simulink model "DIPC4M"  (R2015a)
settings: Solver=ode3  SolverMode=SingleTasking  StartTime=0.0  StopTime=3  FixedStep=1e-3  RelTol=1e-7
values from neighbouring files (symbols this model uses):
  alpha = 1.5    [CaViInit.m]    (also in CaccavaleVillani.m = 2)
  d1 = 1000    [CaViInit.m]    (also in CaccavaleVillani.m = 100)
  delta1 = 80    [CaViInit.m]    (also in CaccavaleVillani.m = 100)
  deltao = 10    [CaViInit.m]    (also in CaccavaleVillani.m = 2000)
  Do = 1500    [CaViInit.m]    (also in CaccavaleVillani.m = 2000)
  g = [0;0;-9.81]    [CaViInit.m]    (also in CaccavaleVillani.m)
  j0 = 0.2    [CaViInit.m]    (also in CaccavaleVillani.m = 1)
  j1 = 2    [CaViInit.m]    (also in CaccavaleVillani.m = 1)
  j1d = 1.00*j1    (= 2)    [CaViInit.m]    (also in CaccavaleVillani.m = 1)
  j2 = 2    [CaViInit.m]    (also in CaccavaleVillani.m = 1)
  j2d = 1.00*j2    (= 2)    [CaViInit.m]    (also in CaccavaleVillani.m = 1)
  j3 = 2    [CaViInit.m]    (also in CaccavaleVillani.m = 1)
  j3d = 1.00*j3    (= 2)    [CaViInit.m]    (also in CaccavaleVillani.m = 1)
  j4 = 2    [CaViInit.m]    (also in CaccavaleVillani.m = 1)
  j4d = 1.00*j4    (= 2)    [CaViInit.m]    (also in CaccavaleVillani.m = 1)
  k1 = 400    [CaViInit.m]    (also in CaccavaleVillani.m = 10000)
  K_o = 700    [CaViInit.m]    (also in CaccavaleVillani.m = 10000)
  kappa1 = 2    [CaViInit.m]    (also in CaccavaleVillani.m = 250)
  kappa_o = 5    [CaViInit.m]    (also in CaccavaleVillani.m = 10000)
  kpr = 150    [CaViInit.m]    (also in CaccavaleVillani.m = 10000)
  kpt = 50    [CaViInit.m]    (also in CaccavaleVillani.m = 50000)
  kv = 300    [CaccavaleVillani.m]
  m0 = 1.4    [CaViInit.m]    (also in CaccavaleVillani.m = 10)
  m1 = 2    [CaViInit.m]    (also in CaccavaleVillani.m = 10)
  m1d = 1.00*m1    (= 2)    [CaViInit.m]    (also in CaccavaleVillani.m = 10)
  m2 = 2    [CaViInit.m]    (also in CaccavaleVillani.m = 10)
  m2d = 1.00*m2    (= 2)    [CaViInit.m]    (also in CaccavaleVillani.m = 10)
  m3 = 2    [CaViInit.m]    (also in CaccavaleVillani.m = 10)
  m3d = 1.00*m3    (= 2)    [CaViInit.m]    (also in CaccavaleVillani.m = 10)
  m4 = 2    [CaViInit.m]    (also in CaccavaleVillani.m = 10)
  m4d = 1.00*m4    (= 2)    [CaViInit.m]    (also in CaccavaleVillani.m = 10)
  r = 0.4*[1; 0; 0 ... (first row only)    [CaViInit.m]    (also in CaccavaleVillani.m = [1; 0; 0)
libraries: aerolibutil x24, dspinverses x3, aerolibtransform2 x2, simulink x2
(part 2 of 2)

== matlab function DIPC4M/Impedance control/Reduced Constraint Matrix ==
  data: r parameter; Ared output; x input
function Ared = ReducedConstraintMAtrix(r,x)
%x_o = [eye(3) zeros(3,4) eye(3) zeros(3,4) eye(3) zeros(3,4) eye(3) zeros(3,4)] * x;
Ared = [-eye(3) skew_sm(quatrot(x(4:7),r(4:6)-r(1:3))) eye(3) zeros(3,15);
        zeros(3) -eye(3) zeros(3) eye(3) zeros(3,12);
        -eye(3) skew_sm(quatrot(x(4:7),r(7:9)-r(1:3))) zeros(3,6) eye(3) zeros(3,9);
        zeros(3) -eye(3) zeros(3,9) eye(3) zeros(3,6);
        -eye(3) skew_sm(quatrot(x(4:7),r(10:12)-r(1:3))) zeros(3,12) eye(3) zeros(3);
        zeros(3) -eye(3) zeros(3,15) eye(3)];
% Ared = [-eye(3) skew_sm(quatrot(x(4:7),x(8:10)-x(1:3))) eye(3) zeros(3,15);
%         zeros(3) -eye(3) zeros(3) eye(3) zeros(3,12);
%         -eye(3) skew_sm(quatrot(x(4:7),x(15:17)-x(1:3))) zeros(3,6) eye(3) zeros(3,9);
%         zeros(3) -eye(3) zeros(3,9) eye(3) zeros(3,6);
%         -eye(3) skew_sm(quatrot(x(4:7),x(22:24)-x(1:3))) zeros(3,12) eye(3) zeros(3);
%         zeros(3) -eye(3) zeros(3,15) eye(3)];

== matlab function DIPC4M/Interaction dynamics1/MATLAB Function ==
  data: r parameter; A output; x input
function A = ConstraintMatrix(r,x)
A = [-eye(3) skew_sm(quatrot(x(4:7),r(1:3))) eye(3) zeros(3,21);
        zeros(3) -eye(3) zeros(3) eye(3) zeros(3,18);
        -eye(3) skew_sm(quatrot(x(4:7),r(4:6))) zeros(3,6) eye(3) zeros(3,15);
        zeros(3) -eye(3) zeros(3,9) eye(3) zeros(3,12);
        -eye(3) skew_sm(quatrot(x(4:7),r(7:9))) zeros(3,12) eye(3) zeros(3,9);
        zeros(3) -eye(3) zeros(3,15) eye(3) zeros(3,6);
        -eye(3) skew_sm(quatrot(x(4:7),r(10:12))) zeros(3,18) eye(3) zeros(3);
        zeros(3) -eye(3) zeros(3,21) eye(3)];

== matlab function DIPC4M/Interaction dynamics1/Centripetal Force ==
  data: dx input; b output; r parameter; x input
function b = centripetalforce(dx,r,x)
b = [skew_sm(dx(4:6))*skew_sm(dx(4:6))*quatrot(x(4:7),r(1:3));
     zeros(3,1);
     skew_sm(dx(4:6))*skew_sm(dx(4:6))*quatrot(x(4:7),r(4:6));
     zeros(3,1);
     skew_sm(dx(4:6))*skew_sm(dx(4:6))*quatrot(x(4:7),r(7:9));
     zeros(3,1);
     skew_sm(dx(4:6))*skew_sm(dx(4:6))*quatrot(x(4:7),r(10:12));
     zeros(3,1)];

== matlab function DIPC4M/Interaction dynamics1/Coriolis Force ==
  data: dx input; hcoriolis output; j0 parameter; m0 parameter
function hcoriolis = CoriolisForce(dx,j0,m0)
hcoriolis = [m0*skew_sm(dx(4:6))*dx(1:3);
        j0*skew_sm(dx(4:6))*dx(4:6)];

== matlab function DIPC4M/Impedance control/Manipulator 2/k1; 2kappa1*eta2 ==
  data: eta1 input; K output; k1 parameter; kappa1 parameter
function K = stiffness(eta1,k1,kappa1)
K = blkdiag(k1*eye(3),2*eta1*kappa1*eye(3));

== matlab function DIPC4M/Impedance control/Manipulator 3/k1; 2kappa1*eta3 ==
  data: eta1 input; K output; k1 parameter; kappa1 parameter
function K = stiffness(eta1,k1,kappa1)
K = blkdiag(k1*eye(3),2*eta1*kappa1*eye(3));

== matlab function DIPC4M/Impedance control/Manipulator 4/k1; 2kappa1*eta4 ==
  data: eta1 input; K output; k1 parameter; kappa1 parameter
function K = stiffness(eta1,k1,kappa1)
K = blkdiag(k1*eye(3),2*eta1*kappa1*eye(3));

== matlab function DIPC4M/Reference Trajectory/VIrtual Object Dynamics/Coriolis Force ==
  data: dx_do input; hcoriolis output; j0 parameter; m0 parameter
function hcoriolis = CoriolisForce(dx_do,j0,m0)
hcoriolis = [m0*skew_sm(dx_do(4:6))*dx_do(1:3);
        j0*skew_sm(dx_do(4:6))*dx_do(4:6)];

== matlab function DIPC4M/Positional Control/Subsystem/Subsystem/k1; 2kappa1*eta1 ==
  data: eta1 input; kpt parameter; kpr parameter; K output
function K = stiffness(eta1,kpt,kpr)
K = blkdiag(kpt*eye(3),2*eta1*kpr*eye(3));

== matlab function DIPC4M/Positional Control/Subsystem/Subsystem1/k1; 2kappa1*eta2 ==
  data: eta2 input; kpt parameter; K output; kpr parameter
function K = stiffness(eta2,kpt,kpr)
K = blkdiag(kpt*eye(3),2*eta2*kpr*eye(3));

== matlab function DIPC4M/Positional Control/Subsystem/Subsystem2/k1; 2kappa1*eta3 ==
  data: eta3 input; kpt parameter; K output; kpr parameter
function K = stiffness(eta3,kpt,kpr)
K = blkdiag(kpt*eye(3),2*eta3*kpr*eye(3));

== matlab function DIPC4M/Positional Control/Subsystem/Subsystem3/k1; 2kappa1*eta4 ==
  data: eta4 input; kpt parameter; K output; kpr parameter
function K = stiffness(eta4,kpt,kpr)
K = blkdiag(kpt*eye(3),2*eta4*kpr*eye(3));

== matlab function DIPC4M/Kinematic Coordination/Grasp Matrix ==
  data: r parameter; G output; x input
function G = GraspMatrix(r,x)
%x_o = [eye(3) zeros(3,4) eye(3) zeros(3,4) eye(3) zeros(3,4) eye(3) zeros(3,4)] * x;
G = [eye(3) zeros(3) eye(3) zeros(3) eye(3) zeros(3) eye(3) zeros(3);
    skew_sm(quatrot(x(4:7),r(1:3))) eye(3) skew_sm(quatrot(x(4:7),r(4:6))) eye(3) skew_sm(quatrot(x(4:7),r(7:9))) eye(3) skew_sm(quatrot(x(4:7),r(10:12))) eye(3)];

== matlab function DIPC4M/Kinematic Coordination/Manipulator Position//Orientation in World Frame ==
  data: p_do input size=3; q_do input size=4; x_d output; r parameter
function x_d = manipulatorpose(p_do,q_do,r)

x_d = [p_do + quatrot(q_do,r(1:3));
        q_do;
        p_do + quatrot(q_do,r(4:6));
        q_do;
        p_do + quatrot(q_do,r(7:9));
        q_do;
        p_do + quatrot(q_do,r(10:12));
        q_do];

== matlab function DIPC4M/Kinematic Coordination/Centripetal Force ==
  data: dx_do input; b output; x input; r parameter
function b = centripetalforce(dx_do,x,r)
%x_o = [eye(3) zeros(3,4) eye(3) zeros(3,4) eye(3) zeros(3,4) eye(3) zeros(3,4)] * x;
b = [skew_sm(dx_do(4:6))*skew_sm(dx_do(4:6))*quatrot(x(4:7),r(1:3));
     zeros(3,1);
     skew_sm(dx_do(4:6))*skew_sm(dx_do(4:6))*quatrot(x(4:7),r(4:6));
     zeros(3,1);
     skew_sm(dx_do(4:6))*skew_sm(dx_do(4:6))*quatrot(x(4:7),r(7:9));
     zeros(3,1);
     skew_sm(dx_do(4:6))*skew_sm(dx_do(4:6))*quatrot(x(4:7),r(10:12));
     zeros(3,1)];

== matlab function DIPC4M/Impedance control/Manipulator 1/k1; 2kappa1*eta1 ==
  data: eta1 input; K output; k1 parameter; kappa1 parameter
function K = stiffness(eta1,k1,kappa1)
K = blkdiag(k1*eye(3),2*eta1*kappa1*eye(3));

== matlab function DIPC4M/Manipulator dynamics/Reduced Constraint Matrix ==
  data: r parameter; Ared output; x input
function Ared = ReducedConstraintMAtrix(r,x)
%x_o = [eye(3) zeros(3,4) eye(3) zeros(3,4) eye(3) zeros(3,4) eye(3) zeros(3,4)] * x;
Ared = [-eye(3) skew_sm(quatrot(x(4:7),r(4:6)-r(1:3))) eye(3) zeros(3,15);
        zeros(3) -eye(3) zeros(3) eye(3) zeros(3,12);
        -eye(3) skew_sm(quatrot(x(4:7),r(7:9)-r(1:3))) zeros(3,6) eye(3) zeros(3,9);
        zeros(3) -eye(3) zeros(3,9) eye(3) zeros(3,6);
        -eye(3) skew_sm(quatrot(x(4:7),r(10:12)-r(1:3))) zeros(3,12) eye(3) zeros(3);
        zeros(3) -eye(3) zeros(3,15) eye(3)];
% Ared = [-eye(3) skew_sm(quatrot(x(4:7),x(8:10)-x(1:3))) eye(3) zeros(3,15);
%         zeros(3) -eye(3) zeros(3) eye(3) zeros(3,12);
%         -eye(3) skew_sm(quatrot(x(4:7),x(15:17)-x(1:3))) zeros(3,6) eye(3) zeros(3,9);
%         zeros(3) -eye(3) zeros(3,9) eye(3) zeros(3,6);
%         -eye(3) skew_sm(quatrot(x(4:7),x(22:24)-x(1:3))) zeros(3,12) eye(3) zeros(3);
%         zeros(3) -eye(3) zeros(3,15) eye(3)];

== matlab function DIPC4M/Manipulator dynamics/Centripal Force ==
  data: r parameter; x input; bred output; dx input
function bred = ReducedCentripetalvector(r,x,dx)
bred = [skew_sm(dx(4:6))*skew_sm(dx(4:6))*quatrot(x(4:7),(r(4:6)-r(1:3)));
        zeros(3,1);
        skew_sm(dx(4:6))*skew_sm(dx(4:6))*quatrot(x(4:7),(r(7:9)-r(1:3)));
        zeros(3,1);
        skew_sm(dx(4:6))*skew_sm(dx(4:6))*quatrot(x(4:7),(r(10:12)-r(1:3)));
        zeros(3,1)];
%     bred = [skew_sm(dx(4:6))*skew_sm(dx(4:6))*quatrot(x(4:7),(x(8:10)-x(1:3)));
%         zeros(3,1);
%         skew_sm(dx(4:6))*skew_sm(dx(4:6))*quatrot(x(4:7),(x(15:17)-x(1:3)));
%         zeros(3,1);
%         skew_sm(dx(4:6))*skew_sm(dx(4:6))*quatrot(x(4:7),(x(22:24)-x(1:3)));
%         zeros(3,1)];

== matlab function DIPC4M/Interaction dynamics/Apparent Inertia ==
  data: G input; Mapp output; M input; m0 parameter; j0 parameter
function Mapp = ApparentInertia(G,M,m0,j0)
Mapp = blkdiag(m0*eye(3),j0*eye(3)) + G*M*G';

== matlab function DIPC4M/Interaction dynamics/Grasp Matrix ==
  data: r parameter; G output; x input
function G = GraspMatrix(r,x)
G = [eye(3) zeros(3) eye(3) zeros(3) eye(3) zeros(3) eye(3) zeros(3);
    skew_sm(quatrot(x(4:7),r(1:3))) eye(3) skew_sm(quatrot(x(4:7),r(4:6))) eye(3) skew_sm(quatrot(x(4:7),r(7:9))) eye(3) skew_sm(quatrot(x(4:7),r(10:12))) eye(3)];

== matlab function DIPC4M/Interaction dynamics/Coriolis Force ==
  data: dx input; hcoriolis output; j0 parameter; m0 parameter
function hcoriolis = CoriolisForce(dx,j0,m0)
hcoriolis = [m0*skew_sm(dx(4:6))*dx(1:3);
        j0*skew_sm(dx(4:6))*dx(4:6)];

== matlab function DIPC4M/Interaction dynamics/Centripetal Force ==
  data: dx input; b output; r parameter; x input
function b = centripetalforce(dx,r,x)
b = [skew_sm(dx(4:6))*skew_sm(dx(4:6))*quatrot(x(4:7),r(1:3));
     zeros(3,1);
     skew_sm(dx(4:6))*skew_sm(dx(4:6))*quatrot(x(4:7),r(4:6));
     zeros(3,1);
     skew_sm(dx(4:6))*skew_sm(dx(4:6))*quatrot(x(4:7),r(7:9));
     zeros(3,1);
     skew_sm(dx(4:6))*skew_sm(dx(4:6))*quatrot(x(4:7),r(10:12));
     zeros(3,1)];

== matlab function DIPC4M/Manipulator motion/Grasp Matrix ==
  data: r parameter; G output; x input
function G = GraspMatrix(r,x)
G = [eye(3) zeros(3) eye(3) zeros(3) eye(3) zeros(3) eye(3) zeros(3);
    skew_sm(quatrot(x(4:7),r(1:3))) eye(3) skew_sm(quatrot(x(4:7),r(4:6))) eye(3) skew_sm(quatrot(x(4:7),r(7:9))) eye(3) skew_sm(quatrot(x(4:7),r(10:12))) eye(3)];

== matlab function DIPC4M/Manipulator motion/Manipualtor pose in world frame ==
  data: p_o input; q_o input size=4; x output; r parameter
function x = manipulatorpose(p_o,q_o,r)

x = [p_o + quatrot(q_o,r(1:3));
        q_o;
        p_o + quatrot(q_o,r(4:6));
        q_o;
        p_o + quatrot(q_o,r(7:9));
        q_o;
        p_o + quatrot(q_o,r(10:12));
        q_o ];

== matlab function DIPC4M/Allocator/MATLAB Function1 ==
  data: r parameter; bred output; dx input; x input
function bred = ReducedCentripetalvector(r,dx,x)
% bred = [skew_sm(dx(4:6))*skew_sm(dx(4:6))*quatrot(x(4:7),r(4:6)-r(1:3));
%     zeros(3,1);
%     skew_sm(dx(4:6))*skew_sm(dx(4:6))*quatrot(x(4:7),r(7:9)-r(1:3));
%     zeros(3,1);
%     skew_sm(dx(4:6))*skew_sm(dx(4:6))*quatrot(x(4:7),r(10:12)-r(1:3));
%     zeros(3,1)];
    bred = [skew_sm(dx(4:6))*skew_sm(dx(4:6))*quatrot(x(4:7),(x(8:10)-x(1:3)));
        zeros(3,1);
        skew_sm(dx(4:6))*skew_sm(dx(4:6))*quatrot(x(4:7),(x(15:17)-x(1:3)));
        zeros(3,1);
        skew_sm(dx(4:6))*skew_sm(dx(4:6))*quatrot(x(4:7),(x(22:24)-x(1:3)));
        zeros(3,1)];

== matlab function DIPC4M/Allocator/MATLAB Function ==
  data: r parameter; Ared output; x input
function Ared = ReducedConstraintMAtrix(r,x)
% Ared = [-eye(3) skew_sm(quatrot(x(4:7),r(4:6)-r(1:3))) eye(3) zeros(3,15);
%         zeros(3) -eye(3) zeros(3) eye(3) zeros(3,12);
%         -eye(3) skew_sm(quatrot(x(4:7),r(7:9)-r(1:3))) zeros(3,6) eye(3) zeros(3,9);
%         zeros(3) -eye(3) zeros(3,9) eye(3) zeros(3,6);
%         -eye(3) skew_sm(quatrot(x(4:7),r(10:12)-r(1:3))) zeros(3,12) eye(3) zeros(3);
%         zeros(3) -eye(3) zeros(3,15) eye(3)];
Ared = [-eye(3) skew_sm(quatrot(x(4:7),x(8:10)-x(1:3))) eye(3) zeros(3,15);
        zeros(3) -eye(3) zeros(3) eye(3) zeros(3,12);
        -eye(3) skew_sm(quatrot(x(4:7),x(15:17)-x(1:3))) zeros(3,6) eye(3) zeros(3,9);
        zeros(3) -eye(3) zeros(3,9) eye(3) zeros(3,6);
        -eye(3) skew_sm(quatrot(x(4:7),x(22:24)-x(1:3))) zeros(3,12) eye(3) zeros(3);
        zeros(3) -eye(3) zeros(3,15) eye(3)];

== matlab function DIPC4M/Manipulator dynamics/World to Object Frame ==
  data: hw input; x input; h_int output
function h_int = inertial2objectFrame(hw,x)

h_int = [quatrot(quatconj(x(4:7)')',hw(1:3));
         hw(4:6);%quatrot(quatconj(x(4:7)')',hw(4:6));
         quatrot(quatconj(x(4:7)')',hw(7:9));
         hw(10:12);%quatrot(quatconj(x(4:7)')',hw(10:12));
         quatrot(quatconj(x(4:7)')',hw(13:15));
         hw(16:18);%quatrot(quatconj(x(4:7)')',hw(16:18));
         quatrot(quatconj(x(4:7)')',hw(19:21));
         hw(22:24)];%quatrot(quatconj(x(4:7)')',hw(22:24));];
